simulink model "Skyhook"  (R2018a)
settings: Solver=VariableStepAuto  StartTime=0.0  StopTime=30  RelTol=1e-3
values from neighbouring files (symbols this model uses):
  cp = 0.8    [Workspace.m]
  kp = 6.32    [Workspace.m]
  ks = 0.0632    [Workspace.m]
  mp = 0.16    [Workspace.m]
  ms = 0.16    [Workspace.m]
  sinefreq = w/2    [Workspace.m]
  T = 0.1450    (= 0.145)    [Workspace.m]
settings Model: Creator=c_s  LastModifiedBy=c_s

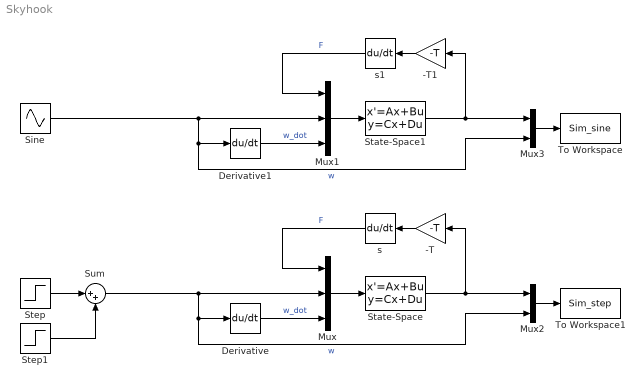
== system Skyhook ==
  -T : Gain  Gain=-T
  -T1 : Gain  Gain=-T
  Derivative : Derivative
  Derivative1 : Derivative
  Mux : Mux  Inputs=3
  Mux1 : Mux  Inputs=3
  Mux2 : Mux  Inputs=2
  Mux3 : Mux  Inputs=2
  Sine : Sin  Amplitude=0.05  Frequency=sinefreq  SampleTime=0
  State-Space : StateSpace  A=[0 1 0 0;-ks/ms 0 ks/ms 0;0 0 0 1;ks/mp 0 -(ks+kp)/mp -cp/mp]  B=[0 0 0;1/ms 0 0;0 0 0;-1/mp kp/mp cp/mp]  C=[1 0 0 0]  D=[0 0 0]  InitialCondition=0
  State-Space1 : StateSpace  A=[0 1 0 0;-ks/ms 0 ks/ms 0;0 0 0 1;ks/mp 0 -(ks+kp)/mp -cp/mp]  B=[0 0 0;1/ms 0 0;0 0 0;-1/mp kp/mp cp/mp]  C=[1 0 0 0]  D=[0 0 0]  InitialCondition=0
  Step : Step  After=0.05  SampleTime=0
  Step1 : Step  Time=2  After=-0.05  SampleTime=0
  Sum : Sum  Inputs=|++
  To Workspace : ToWorkspace  VariableName=Sim_sine  SaveFormat=Structure With Time  SampleTime=-1
  To Workspace1 : ToWorkspace  VariableName=Sim_step  SaveFormat=Structure With Time  SampleTime=-1
  s : Derivative
  s1 : Derivative
  wires:
  State-Space/1 -> -T/1, Mux2/1
  s/1 -> Mux/1  "F"
  Mux/1 -> State-Space/1
  -T/1 -> s/1
  Step1/1 -> Sum/2
  Step/1 -> Sum/1
  Sum/1 -> Mux2/2, Derivative/1, Mux/2  "w"
  Derivative/1 -> Mux/3  "w_dot"
  Sine/1 -> Mux3/2, Derivative1/1, Mux1/2  "w"
  Mux1/1 -> State-Space1/1
  State-Space1/1 -> Mux3/1, -T1/1
  -T1/1 -> s1/1
  Derivative1/1 -> Mux1/3  "w_dot"
  s1/1 -> Mux1/1  "F"
  Mux2/1 -> To Workspace1/1
  Mux3/1 -> To Workspace/1
